simulink model "hw3_b_ELS_model_c05"  (R2024b)
settings: Solver=ode4  StartTime=0.0  StopTime=sim_time*10  FixedStep=sample_time  RelTol=1e-3
values from neighbouring files (symbols this model uses):
  a = -0.8    [hw3_a_rls_v2.m]    (also in hw3_b_rls_v2.m)
  b = 0.5    [hw3_a_rls_v2.m]    (also in hw3_b_rls_v2.m)
  c = -0.5    [hw3_a_rls_v2.m]    (also in hw3_b_rls_v2.m = 0)
  noise_mean = 0    [hw3_a_rls_v2.m]    (also in hw3_b_rls_v2.m)
  noise_seed = round(rand*1e5)    [hw3_a_rls_v2.m]    (also in hw3_b_rls_v2.m)
  noise_variance = 0.5    [hw3_a_rls_v2.m]    (also in hw3_b_rls_v2.m)
  P_0 = eye(3,3) * 100    [hw3_a_rls_v2.m]    (also in hw3_b_rls_v2.m)
  phi_0 = zeros(3,1)    [hw3_b_rls_v2.m]
  sample_time = 1    [hw3_a_rls_v2.m]    (also in hw3_b_rls_v2.m)
  Theta_0 = [0;0;0]    [hw3_a_rls_v2.m]    (also in hw3_b_rls_v2.m)
libraries: simulink x1
settings Model: Creator=kemal  LastModifiedBy=kemal

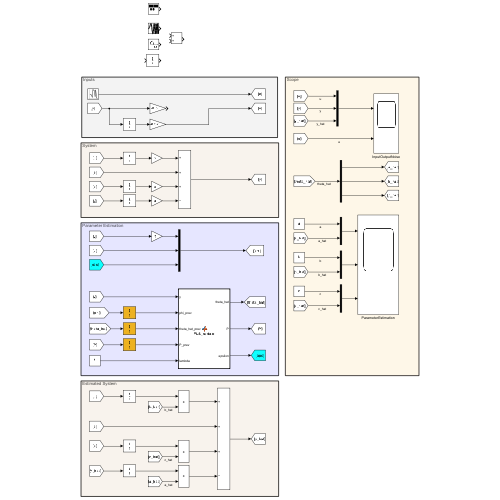
[thumbnail: Simulink's stored preview of the top-level diagram]
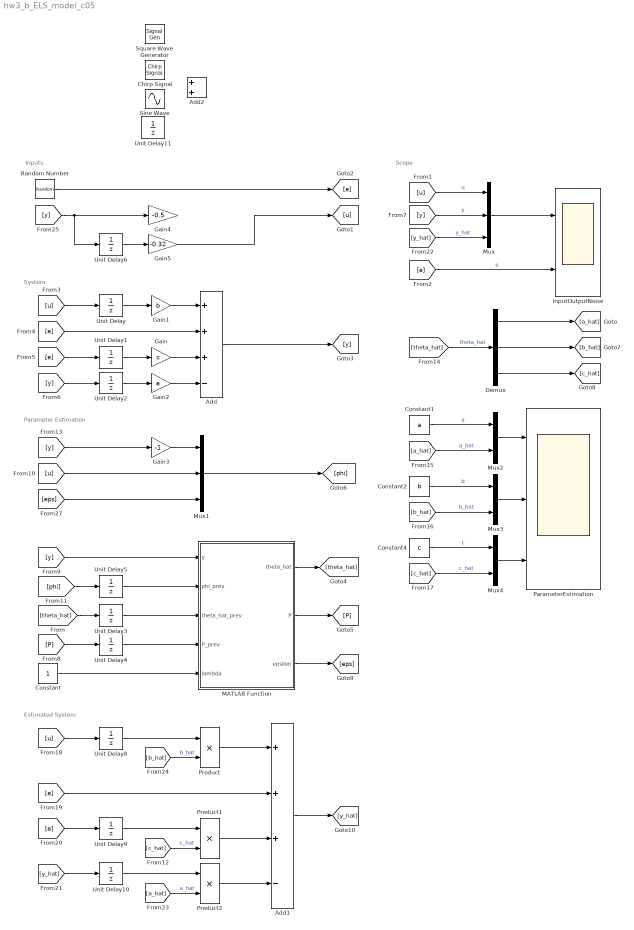
== system hw3_b_ELS_model_c05 ==
  note: System
  note: Scope
  note: Parameter Estimation
  note: Estimated System
  note: Inputs
  Add : Sum  Inputs=+++-
  Add1 : Sum  Inputs=+++-
  Add2 : Sum
  Chirp Signal : simulink/Sources/Chirp Signal  f1=0.1  T=100  f2=1000
  Constant : Constant  SampleTime=-1
  Constant1 : Constant  Value=a  SampleTime=sample_time
  Constant2 : Constant  Value=b  SampleTime=sample_time
  Constant4 : Constant  Value=c  SampleTime=sample_time
  Demux : Demux  Outputs=3
  Gain : Gain  Gain=c
  Gain1 : Gain  Gain=b
  Gain2 : Gain  Gain=a
  Gain3 : Gain  Gain=-1
  Gain4 : Gain  Gain=-0.5
  Gain5 : Gain  Gain=-0.32
  InputOutputNoise : Scope  NumInputPorts=2
  MATLAB Function : MATLAB Function  TreatAsAtomicUnit=on
  Mux : Mux  Inputs=3
  Mux1 : Mux  Inputs=3
  Mux2 : Mux  Inputs=2
  Mux3 : Mux  Inputs=2
  Mux4 : Mux  Inputs=2
  ParameterEstimation : Scope  NumInputPorts=3
  Product : Product
  Product1 : Product
  Product2 : Product
  Random Number : RandomNumber  Mean=noise_mean  Variance=noise_variance  Seed=noise_seed  SampleTime=sample_time
  Sine Wave : Sin  Amplitude=5  Frequency=2*pi/10  SampleTime=0
  Square Wave Generator : SignalGenerator  WaveForm=square  Frequency=1/100
  Unit Delay{,1..2,6,8..11} (8 alike) : UnitDelay  SampleTime=sample_time  HasFrameUpgradeWarning=on
  Unit Delay3 : UnitDelay  InitialCondition=Theta_0  SampleTime=sample_time  HasFrameUpgradeWarning=on
  Unit Delay4 : UnitDelay  InitialCondition=P_0  SampleTime=sample_time  HasFrameUpgradeWarning=on
  Unit Delay5 : UnitDelay  InitialCondition=phi_0  SampleTime=sample_time  HasFrameUpgradeWarning=on
  wires:
  [u] -> Unit Delay/1
  [e] -> Unit Delay1/1
  Unit Delay1/1 -> Gain/1
  Unit Delay/1 -> Gain1/1
  Gain/1 -> Add/3
  [e] -> Add/2
  Gain1/1 -> Add/1
  [y] -> Unit Delay2/1
  Unit Delay2/1 -> Gain2/1
  Gain2/1 -> Add/4
  Add/1 -> [y]
  [u] -> Mux/1  "u"
  [y] -> Mux/2  "y"
  [e] -> InputOutputNoise/2  "e"
  Mux/1 -> InputOutputNoise/1
  MATLAB Function/2(P) -> [P]
  MATLAB Function/1(theta_hat) -> [theta_hat]
  [theta_hat] -> Unit Delay3/1
  Unit Delay3/1 -> MATLAB Function/3(theta_hat_prev)
  [P] -> Unit Delay4/1
  Unit Delay4/1 -> MATLAB Function/4(P_prev)
  Constant/1 -> MATLAB Function/5(lambda)
  [y] -> Gain3/1
  Gain3/1 -> Mux1/1
  Mux1/1 -> [phi]
  [phi] -> Unit Delay5/1
  [theta_hat] -> Demux/1  "theta_hat"
  Mux2/1 -> ParameterEstimation/1
  Mux3/1 -> ParameterEstimation/2
  Constant1/1 -> Mux2/1  "a"
  Demux/1 -> [a_hat]
  Demux/2 -> [b_hat]
  Constant2/1 -> Mux3/1  "b"
  [a_hat] -> Mux2/2  "a_hat"
  [b_hat] -> Mux3/2  "b_hat"
  [y_hat] -> Mux/3  "y_hat"
  [u] -> Mux1/2
  Unit Delay5/1 -> MATLAB Function/2(phi_prev)
  Constant4/1 -> Mux4/1  "c"
  Mux4/1 -> ParameterEstimation/3
  Demux/3 -> [c_hat]
  [c_hat] -> Mux4/2  "c_hat"
  MATLAB Function/3(epsilon) -> [eps]
  [e] -> Add1/2
  Unit Delay10/1 -> Product2/1
  [a_hat] -> Product2/2  "a_hat"
  [c_hat] -> Product1/2  "c_hat"
  [b_hat] -> Product/2  "b_hat"
  Product2/1 -> Add1/4
  Unit Delay9/1 -> Product1/1
  Product1/1 -> Add1/3
  Product/1 -> Add1/1
  [u] -> Unit Delay8/1
  [e] -> Unit Delay9/1
  Unit Delay8/1 -> Product/1
  [y_hat] -> Unit Delay10/1
  Add1/1 -> [y_hat]
  [y] -> Unit Delay6/1, Gain4/1
  Random Number/1 -> [e]
  Unit Delay6/1 -> Gain5/1
  [y] -> MATLAB Function/1(y)
  [eps] -> Mux1/3
  Gain5/1 -> [u]

== matlab function hw3_b_ELS_model_c05/MATLAB Function ==
  data: y input; theta_hat output; phi_prev input; theta_hat_prev input; P_prev input; lambda input; P output; epsilon output
function [theta_hat, P, epsilon] = RLS_update(y, phi_prev, theta_hat_prev, P_prev, lambda)
    % Compute innovation
    epsilon = y - phi_prev' * theta_hat_prev;
     
    % Update covariance matrix
    P = (1/lambda) * (P_prev - (P_prev * (phi_prev * phi_prev') * P_prev) / ...
        (lambda + phi_prev' * P_prev * phi_prev));

    % Update parameter estimate
    theta_hat = theta_hat_prev + P * phi_prev * epsilon;
end
